simulink model "initial_Test"  (R2019a)
settings: Solver=VariableStepAuto  StartTime=0.0  StopTime=1  RelTol=1e-3
settings Model: Creator=Yusuf  LastModifiedBy=Yusuf

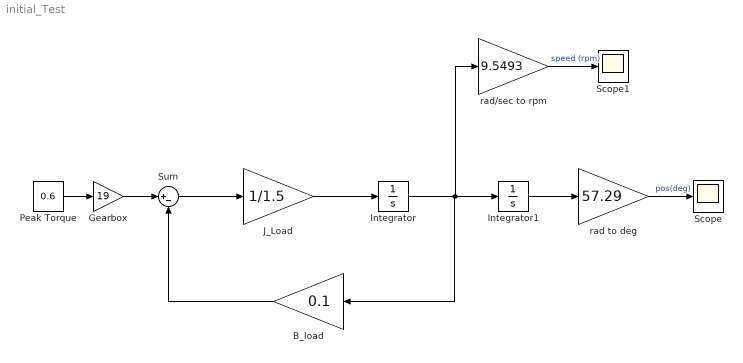
== system initial_Test ==
  B_load : Gain  Gain=0.1
  Gearbox : Gain  Gain=19
  Integrator : Integrator
  Integrator1 : Integrator
  J_Load : Gain  Gain=1/1.5
  Peak Torque : Constant  Value=0.6
  Scope : Scope
  Scope1 : Scope
  Sum : Sum  Inputs=|+-
  rad to deg : Gain  Gain=57.29
  rad/sec to rpm : Gain  Gain=9.5493
  wires:
  Sum/1 -> J_Load/1
  J_Load/1 -> Integrator/1
  Integrator/1 -> rad/sec to rpm/1, Integrator1/1, B_load/1
  B_load/1 -> Sum/2
  Integrator1/1 -> rad to deg/1
  rad to deg/1 -> Scope/1  "pos(deg)"
  rad/sec to rpm/1 -> Scope1/1  "speed (rpm)"
  Peak Torque/1 -> Gearbox/1
  Gearbox/1 -> Sum/1
